simulink subsystem "Day6_Scenario_1"  (R2024a)
settings: Solver=VariableStepAuto  StartTime=0.0  StopTime=10.0  RelTol=1e-3
undefined symbols (not defined in the file): route1_waypoint
libraries: CarMaker4SL x15, slpidlib x1
settings Model: Creator=junhyung.cha  LastModifiedBy=User

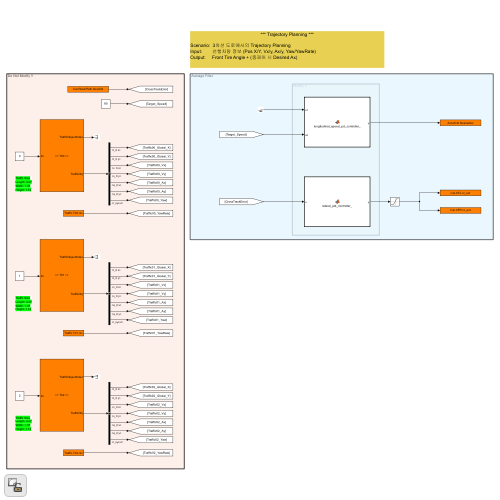
[thumbnail: Simulink's stored preview of the top-level diagram]
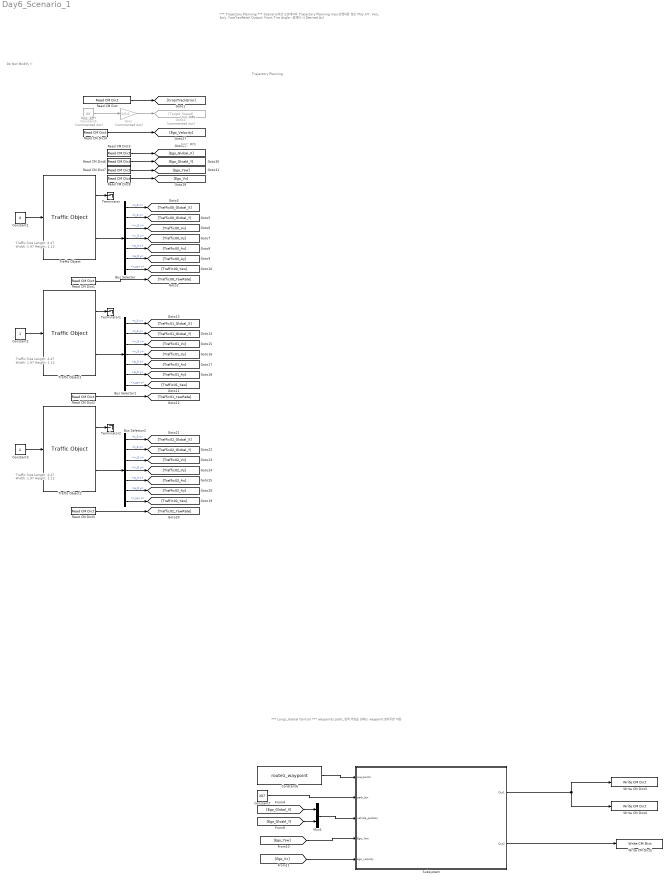
== system Day6_Scenario_1 ==
  note: Do Not Modify !!
  note: Traffic Size
      | Length: 4.47
      | Width: 1.97
      | Height: 1.12
  note: Traffic Size
      | Length: 4.47
      | Width: 1.97
      | Height: 1.12
  note: Traffic Size
      | Length: 4.47
      | Width: 1.97
      | Height: 1.12
  note: *** Trajectory Planning ***
      |
      | Scenario: 3차선 도로에서의 Trajectory Planning
      | Input: 선행차량 정보 (Pos X/Y, Vx/y, Ax/y, Yaw/YawRate)
      | Output: Front Tire Angle + (종제어 시 Desired Ax)
  note: Unit: MPS
  note: Unit: KPH
  note: Unit: MPS
  note: Trajectory Planning
  note: *** Longi_lateral Control ***
      |
      | waypoints
      | path_len
      | 입력 부분을 원하는 waypoint 넣어주면 작동
  Bus Selector : BusSelector  OutputSignals=t_0 x,t_0 y,v_0 x,v_0 y,a_0 x,a_0 y,r_zyx z
  Bus Selector1 : BusSelector  OutputSignals=t_0 x,t_0 y,v_0 x,v_0 y,a_0 x,a_0 y,r_zyx z
  Bus Selector2 : BusSelector  OutputSignals=t_0 x,t_0 y,v_0 x,v_0 y,a_0 x,a_0 y,r_zyx z
  Constant1 : Constant  Value=0
  Constant2 : Constant
  Constant3 : Constant  Value=2
  Constant4 : Constant  Commented=on  Value=80
  Constant6 : Constant  Value=route1_waypoint
  Constant7 : Constant  Value=207
  Gain : Gain  Commented=on  Gain=1/3.6
  Goto4 : Goto  Commented=on  GotoTag=Target_Speed
  Mux1 : Mux  Inputs=2
  Read CM Dict : CarMaker4SL/Read CM Dict  xname=Car.Road.Path.DevDist  xsync=off  xstime=Inherited
  Read CM Dict1 : CarMaker4SL/Read CM Dict  xname=Traffic.T00.rzv  xsync=off  xstime=Inherited
  Read CM Dict2 : CarMaker4SL/Read CM Dict  xname=Traffic.T01.rzv  xsync=off  xstime=Inherited
  Read CM Dict3 : CarMaker4SL/Read CM Dict  xname=Traffic.T02.rzv  xsync=off  xstime=Inherited
  Read CM Dict4 : CarMaker4SL/Read CM Dict  xname=Car.v  xsync=off  xstime=Inherited
  Read CM Dict5 : CarMaker4SL/Read CM Dict  xname=Car.Fr1.tx  xsync=off  xstime=Inherited
  Read CM Dict6 : CarMaker4SL/Read CM Dict  xname=Car.Fr1.ty  xsync=off  xstime=Inherited
  Read CM Dict7 : CarMaker4SL/Read CM Dict  xname=Car.Fr1.rz  xsync=off  xstime=Inherited
  Read CM Dict8 : CarMaker4SL/Read CM Dict  xname=Car.v  xsync=off  xstime=Inherited
  Subsystem : Subsystem
  Terminator : Terminator
  Terminator1 : Terminator
  Terminator2 : Terminator
  Traffic Object : CarMaker4SL/Traffic Object  xname=T00  ximode=Traffic Id  xstime=Inherited
      settings: SourceProductName=CarMaker4SL
  Traffic Object1 : CarMaker4SL/Traffic Object  xname=T01  ximode=Traffic Id  xstime=Inherited
      settings: SourceProductName=CarMaker4SL
  Traffic Object2 : CarMaker4SL/Traffic Object  xname=T02  ximode=Traffic Id  xstime=Inherited
      settings: SourceProductName=CarMaker4SL
  Write CM Dict3 : CarMaker4SL/Write CM Dict  xname=Car.CFL.rz_ext  xsync=off
  Write CM Dict4 : CarMaker4SL/Write CM Dict  xname=Car.CFR.rz_ext  xsync=off
  Write CM Dict5 : CarMaker4SL/Write CM Dict  xname=AccelCtrl.DesiredAx  xsync=off
  wires:
  Constant1/1 -> Traffic Object/1
  Read CM Dict/1 -> [CrossTrackError]
  Gain/1 -> Goto4/1
  Bus Selector/4 -> [Traffic00_Vy]  "<v_0 y>"
  Traffic Object/1 -> Terminator/1
  Bus Selector/3 -> [Traffic00_Vx]  "<v_0 x>"
  Traffic Object/2 -> Bus Selector/1
  Bus Selector/1 -> [Traffic00_Global_X]  "<t_0 x>"
  Bus Selector/2 -> [Traffic00_Global_Y]  "<t_0 y>"
  Read CM Dict1/1 -> [Traffic00_YawRate]
  Bus Selector/5 -> [Traffic00_Ax]  "<a_0 x>"
  Bus Selector/6 -> [Traffic00_Ay]  "<a_0 y>"
  Bus Selector/7 -> [Traffic00_Yaw]  "<r_zyx z>"
  Read CM Dict2/1 -> [Traffic01_YawRate]
  Bus Selector1/1 -> [Traffic01_Global_X]  "<t_0 x>"
  Bus Selector1/5 -> [Traffic01_Ax]  "<a_0 x>"
  Bus Selector1/6 -> [Traffic01_Ay]  "<a_0 y>"
  Bus Selector1/7 -> [Traffic01_Yaw]  "<r_zyx z>"
  Traffic Object1/1 -> Terminator1/1
  Bus Selector1/4 -> [Traffic01_Vy]  "<v_0 y>"
  Constant2/1 -> Traffic Object1/1
  Traffic Object1/2 -> Bus Selector1/1
  Bus Selector1/3 -> [Traffic01_Vx]  "<v_0 x>"
  Bus Selector1/2 -> [Traffic01_Global_Y]  "<t_0 y>"
  Bus Selector2/3 -> [Traffic02_Vx]  "<v_0 x>"
  Bus Selector2/2 -> [Traffic02_Global_Y]  "<t_0 y>"
  Traffic Object2/2 -> Bus Selector2/1
  Bus Selector2/1 -> [Traffic02_Global_X]  "<t_0 x>"
  Bus Selector2/6 -> [Traffic02_Ay]  "<a_0 y>"
  Constant3/1 -> Traffic Object2/1
  Traffic Object2/1 -> Terminator2/1
  Bus Selector2/7 -> [Traffic02_Yaw]  "<r_zyx z>"
  Bus Selector2/5 -> [Traffic02_Ax]  "<a_0 x>"
  Read CM Dict3/1 -> [Traffic02_YawRate]
  Bus Selector2/4 -> [Traffic02_Vy]  "<v_0 y>"
  Read CM Dict4/1 -> [Ego_Velocity]
  Constant4/1 -> Gain/1
  Read CM Dict8/1 -> [Ego_Vx]
  Read CM Dict5/1 -> [Ego_Global_X]
  Read CM Dict6/1 -> [Ego_Gloabl_Y]
  Read CM Dict7/1 -> [Ego_Yaw]
  Constant7/1 -> Subsystem/2(path_len)
  Constant6/1 -> Subsystem/1(waypoints)
  [Ego_Global_X] -> Mux1/1
  [Ego_Gloabl_Y] -> Mux1/2
  Mux1/1 -> Subsystem/3(vehicle_position)
  [Ego_Yaw] -> Subsystem/4(Ego_Yaw)
  [Ego_Vx] -> Subsystem/5(ego_velocity)
  Subsystem/1(Out1) -> Write CM Dict4/1, Write CM Dict3/1
  Subsystem/2(Out2) -> Write CM Dict5/1

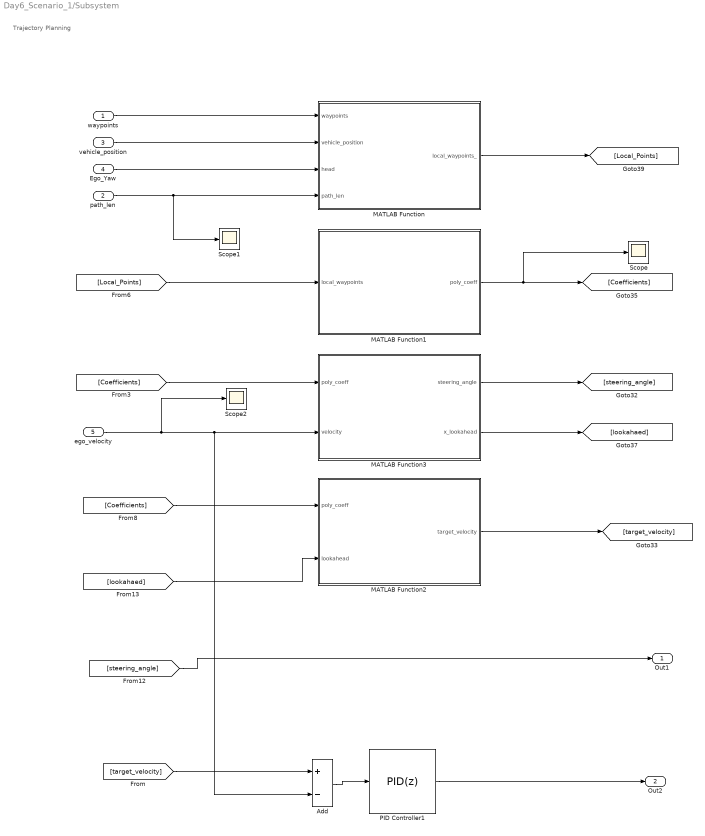
== system Day6_Scenario_1/Subsystem ==
  note: Trajectory Planning
  waypoints : Inport
  path_len : Inport  Port=2
  vehicle_position : Inport  Port=3
  Ego_Yaw : Inport  Port=4
  ego_velocity : Inport  Port=5
  Add : Sum  Inputs=+-
  MATLAB Function : MATLAB Function  TreatAsAtomicUnit=on
  MATLAB Function1 : MATLAB Function  TreatAsAtomicUnit=on
  MATLAB Function2 : MATLAB Function  TreatAsAtomicUnit=on
  MATLAB Function3 : MATLAB Function  TreatAsAtomicUnit=on
  PID Controller1 : slpidlib/PID Controller  Controller=PID  Form=Parallel  TimeDomain=Discrete-time  UseExternalTs=off  SampleTime=-1  IntegratorMethod=Forward Euler  FilterMethod=Forward Euler  ControllerParametersSource=internal  P=3  I=0  UseKiTs=off  D=0.0  UseExternalDerivativeSource=off  N=100  UseFilter=off  TunerSelectOption=Transfer Function Based (PID Tuner App)  InitialConditionSource=internal  InitialConditionForIntegrator=0  InitialConditionForFilter=0  DifferentiatorICPrevScaledInput=0  ExternalReset=none  TrackingMode=off  Kt=1  LimitOutput=off  SatLimitsSource=internal  UpperSaturationLimit=inf  LowerSaturationLimit=-inf  LinearizeAsGain=on  AntiWindupMode=none  Kb=1  LimitIntegrator=off  UpperIntegratorSaturationLimit=inf  LowerIntegratorSaturationLimit=-inf  POutMin=[]  POutMax=[]  IOutMin=[]  IOutMax=[]  DOutMin=[]  DOutMax=[]  NOutMin=[]  NOutMax=[]  SumOutMin=[]  SumOutMax=[]  SaturationOutMin=[]  SaturationOutMax=[]  PParamMin=[]  PParamMax=[]  IParamMin=[]  IParamMax=[]  DParamMin=[]  DParamMax=[]  NParamMin=[]  NParamMax=[]  KbParamMin=[]  KbParamMax=[]  KtParamMin=[]  KtParamMax=[]  KbOutMin=[]  KbOutMax=[]  KtOutMin=[]  KtOutMax=[]  IntegratorOutMin=[]  IntegratorOutMax=[]  FilterOutMin=[]  FilterOutMax=[]  SumI1OutMin=[]  SumI1OutMax=[]  SumI2OutMin=[]  SumI2OutMax=[]  SumI3OutMin=[]  SumI3OutMax=[]  SumI4OutMin=[]  SumI4OutMax=[]  SumDOutMin=[]  SumDOutMax=[]  DifferentiatorOutMin=[]  DifferentiatorOutMax=[]  FilterDiffOutCoefMin=[]  FilterDiffOutCoefMax=[]  ReciprocalOutMin=[]  ReciprocalOutMax=[]  SumDenOutMin=[]  SumDenOutMax=[]  SumNumOutMin=[]  SumNumOutMax=[]  DivideOutMin=[]  DivideOutMax=[]  UdiffTsProdOutMin=[]  UdiffTsProdOutMax=[]  NTsProdOutMin=[]  NTsProdOutMax=[]  UintegralTsProdOutMin=[]  UintegralTsProdOutMax=[]  UngainTsProdOutMin=[]  UngainTsProdOutMax=[]  ClampingZeroOutDataTypeStr=Inherit: Inherit via back propagation  ClampingZeroOutMin=[]  ClampingZeroOutMax=[]  FilterDenConstantOutDataTypeStr=Inherit: Inherit via back propagation  FilterDenConstantOutMin=[]  FilterDenConstantOutMax=[]  PCopyOutDataTypeStr=Inherit: Inherit via back propagation  PCopyOutMin=[]  PCopyOutMax=[]  NCopyOutDataTypeStr=Inherit: Inherit via back propagation  NCopyOutMin=[]  NCopyOutMax=[]  IntegratorContinuousStateAttributes=''  IntegratorStateMustResolveToSignalObject=off  IntegratorRTWStateStorageClass=Auto  FilterContinuousStateAttributes=''  FilterStateMustResolveToSignalObject=off  FilterRTWStateStorageClass=Auto  ParallelPVariant=InternalParameters  IdealPVariant=Disabled  IVariant=InternalParameters  DVariant=InternalParameters  IntegratorVariant=Discrete  SatVariant=Disabled  AWVariant=Passthrough  PCopyVariant=Disabled  TRVariant=Disabled  FdbkBlocksVariant=Forward  IdealPFdbkVariant=Disabled  SatFdbkVariant=Disabled  DerivativeFilterVariant=Differentiator  NVariant=Passthrough  NCopyVariant=Disabled_SignalSpec  FilterICVariant=InternalICsDifferentiator  IntegratorICVariant=InternalICs  ExternalResetVariant=Disabled  TRSumVariant=Passthrough  SumFdbkVariant=Disabled  SumVariant=Sum_PID  TsampFilterVariant=InternalTs  TsampNgainVariant=Passthrough  TsampIntegralVariant=Disabled_SignalSpec  ExternalSaturationOutDataTypeStr=Inherit: Same as second input  DerivativeSourceVariant=ErrorSignal
  Scope : Scope
  Scope1 : Scope
  Scope2 : Scope
  Out1 : Outport
  Out2 : Outport  Port=2
  wires:
  [target_velocity] -> Add/1
  vehicle_position/1 -> MATLAB Function/2(vehicle_position)
  PID Controller1/1 -> Out2/1
  [steering_angle] -> Out1/1
  ego_velocity/1 -> MATLAB Function3/2(velocity), Add/2, Scope2/1
  Ego_Yaw/1 -> MATLAB Function/3(head)
  path_len/1 -> MATLAB Function/4(path_len), Scope1/1
  [lookahaed] -> MATLAB Function2/2(lookahead)
  [Coefficients] -> MATLAB Function2/1(poly_coeff)
  MATLAB Function2/1(target_velocity) -> [target_velocity]
  MATLAB Function1/1(poly_coeff) -> [Coefficients], Scope/1
  [Local_Points] -> MATLAB Function1/1(local_waypoints)
  [Coefficients] -> MATLAB Function3/1(poly_coeff)
  Add/1 -> PID Controller1/1
  MATLAB Function/1(local_waypoints_) -> [Local_Points]
  MATLAB Function3/1(steering_angle) -> [steering_angle]
  MATLAB Function3/2(x_lookahead) -> [lookahaed]
  waypoints/1 -> MATLAB Function/1(waypoints)

== matlab function Day6_Scenario_1/Subsystem/MATLAB Function ==
  data: waypoints input; local_waypoints_ output; vehicle_position input; head input; path_len input
function local_waypoints_ = global_to_local_waypoints(waypoints, vehicle_position, head, path_len)
    % 로컬 좌표 변환 함수 (yaw 변화가 작으면 무시)
    % 입력:
    %   waypoints        : [N x 2] 전체 전역 경로
    %   vehicle_position : [1 x 2] 자차 위치 [x, y]
    %   head             : 자차 yaw [rad]
    %   path_len         : 유효 경로 길이

    local_waypoints_ = zeros(400, 2);  % Simulink 고정 크기 호환

 

    x_ego = vehicle_position(1);
    y_ego = vehicle_position(2);

    waypoints_x = waypoints(:, 1);
    waypoints_y = waypoints(:, 2);

    % --- 전체 경로를 로컬 좌표계로 변환 ---
    for i = 1:path_len
        dx = waypoints_x(i) - x_ego;
        dy = waypoints_y(i) - y_ego;

        x_local = dx * cos(-head) - dy * sin(-head);
        y_local = dx * sin(-head) + dy * cos(-head);

        local_waypoints_(i, :) = [x_local, y_local];
    end
end

== matlab function Day6_Scenario_1/Subsystem/MATLAB Function1 ==
  data: local_waypoints input; poly_coeff output
function poly_coeff = fit_polynomial_to_waypoints(local_waypoints)
% 전방 포인트(x > 0) 중 y값 차이가 10 이하이며, y값이 -30~30 사이인 포인트만 사용

    % 1차 필터링: x > 0
    valid_idx = local_waypoints(:,1) > 0;
    filtered = local_waypoints(valid_idx, :);

    % 2차 필터링: y in [-8, 8]
    y_range_idx = abs(filtered(:,2)) <= 8;
    filtered = filtered(y_range_idx, :);

    % 앞쪽 30개만 사용
    N = min(30, size(filtered, 1));
    x = filtered(1:N, 1);
    y = filtered(1:N, 2);

    % 최소 포인트 수 확인 후 3차 다항식 피팅
    if length(x) >= 4
        poly_coeff = polyfit(x, y, 3);
    else
        poly_coeff = zeros(1, 4);
    end
end

== matlab function Day6_Scenario_1/Subsystem/MATLAB Function2 ==
  data: poly_coeff input; target_velocity output; lookahead input
function target_velocity = longitudinal_speed_control_from_poly(poly_coeff, lookahead)
    V_max = 30.0/3.6;
  
    x_for_curv = lookahead;

    % 곡률 계산
    dy_dx   = polyval(polyder(poly_coeff), x_for_curv);
    d2y_dx2 = polyval(polyder(polyder(poly_coeff)), x_for_curv);
    kappa = d2y_dx2 / (1 + dy_dx^2)^(3/2);



    v_from_curvature = V_max * exp(-5.0 * abs(kappa));
    v = v_from_curvature;


    target_velocity = v;

    % % ======== 저역통과 필터 (optional) =========
    % persistent prev_v
    % if isempty(prev_v)
    %     prev_v = v;
    % end
    % 
    % alpha = 0.95;  % 0.85~0.95 추천 (1에 가까울수록 부드럽고 느림)
    % target_velocity = alpha * prev_v + (1 - alpha) * v;
    % prev_v = target_velocity;
end

== matlab function Day6_Scenario_1/Subsystem/MATLAB Function3 ==
  data: poly_coeff input; steering_angle output; velocity input; x_lookahead output
function [steering_angle, x_lookahead] = adaptive_pure_pursuit_from_poly(poly_coeff, velocity)
% Adaptive Pure Pursuit with dynamic lookahead based on velocity and curvature
% 입력:
%   poly_coeff : 경로 다항식 계수 [1x4] (y = ax^3 + bx^2 + cx + d)
%   velocity   : 자차 속도 [m/s]
% 출력:
%   steering_angle : 조향각 [rad]
%   x_lookahead    : lookahead 거리 [m]

    % 차량 파라미터
    L = 2.9;  % 차량 휠베이스 [m]

    % Lookahead 계산 파라미터
    Lxd = 2.5;       % 기본 lookahead [m]
    kv = 0.8;        % 속도 계수
    kc = 1;       % 곡률 보정 계수
    rad2deg = 180 / pi;

    % 곡률 평가 위치 (예: x=3.0)에서 곡률 추정
    x_for_curv = 3.0;
    dy_dx  = polyval(polyder(poly_coeff), x_for_curv);
    d2y_dx2 = polyval(polyder(polyder(poly_coeff)), x_for_curv);
    curvature = d2y_dx2 / (1 + dy_dx^2)^(3/2);  % 곡률

    % lookahead 거리 계산
    x_lookahead = Lxd + kv * velocity - kc * abs(curvature * rad2deg);
    x_lookahead = max(2.0, x_lookahead);  % 최소 거리 제한

    % lookahead 위치에서 목표점 좌표
    y_target = polyval(poly_coeff, x_lookahead);

    % 좌표 기반 조향각 계산 (Pure Pursuit 방식)
    alpha = atan2(y_target, x_lookahead);  % heading error
    steering_angle = atan2(2 * L * sin(alpha), x_lookahead);


    
end
